simulink model "OPC_prueba_MPC_observador"  (R2018a)
settings: Solver=FixedStepAuto  StartTime=0.0  StopTime=inf  FixedStep=0.1  RelTol=1e-3
values from neighbouring files (symbols this model uses):
  Ad = sysd.A    [SimulinkInit.m]
  Bd = sysd.B    [SimulinkInit.m]
  Cd = sysd.C    [SimulinkInit.m]
libraries: opclib x7, mpclib x2
settings Model: Creator=cmparedes  LastModifiedBy=Diego
settings SolverCC: AutoInsertRateTranBlk=on

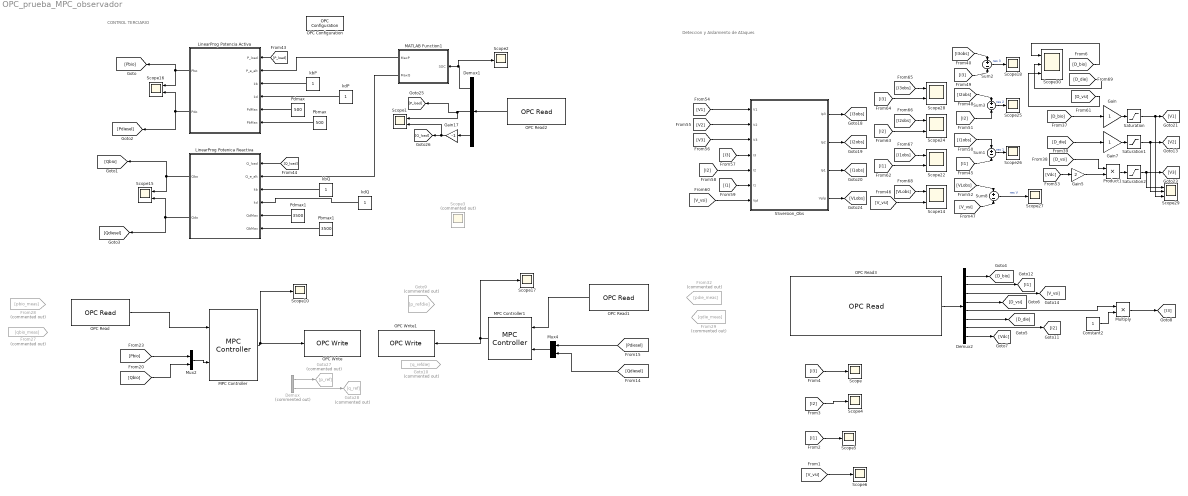
== system OPC_prueba_MPC_observador ==
  note: CONTROL TERCIARIO
  note: Deteccion y Aislamiento de Ataques
  Constant2 : Constant
  Demux : Demux  Commented=on  Outputs=2
  Demux1 : Demux  Outputs=3
  Demux2 : Demux  Outputs=8
  From27 : From  Commented=on  GotoTag=qbio_meas
  From28 : From  Commented=on  GotoTag=pbio_meas
  From29 : From  Commented=on  GotoTag=qdie_meas
  From32 : From  Commented=on  GotoTag=pdie_meas
  Gain : Gain
  Gain17 : Gain  Gain=-1
  Gain5 : Gain  Gain=2
  Gain7 : Gain
  Goto10 : Goto  Commented=on  GotoTag=q_refdie
  Goto27 : Goto  Commented=on  GotoTag=p_ref
  Goto28 : Goto  Commented=on  GotoTag=q_ref
  Goto9 : Goto  Commented=on  GotoTag=p_refdie
  LinearProg Potencia Activa : MATLAB Function  TreatAsAtomicUnit=on  SystemSampleTime=.1
  LinearProg Potenica Reactiva : MATLAB Function  TreatAsAtomicUnit=on  SystemSampleTime=.1
  MATLAB Function1 : MATLAB Function  TreatAsAtomicUnit=on
  MPC Controller : mpclib/MPC Controller  mpcobj=mpcobj  x0=[]  is_multiple=0  enable_value=0  return_u0=off  updateMPCinCallerWorkspace=on  ref_from_ws=off  ref_signal_name=[]  ref_preview=on  md_from_ws=off  md_signal_name=[]  md_preview=on  from_project=off  project_file=MPCtask.mat  md_inport=off  mv_inport=off  cost_outport=off  return_sequence=off  return_qpstatus=off  return_state=off  state_inport=off  lims_inport=off  cc_inport=off  ywt_inport=off  is_designfromscratch=0  uwt_inport=off  duwt_inport=off  rhoeps_inport=off  uref_inport=off  n_ts=0.1  n_p=100  n_mv=2  n_md=0  n_ud=0  n_mo=2  n_uo=0  BlockDataType=double  SampleTimeInherited=off  switch_inport=off
  MPC Controller1 : mpclib/MPC Controller  mpcobj=mpcobj  x0=[]  is_multiple=0  enable_value=0  return_u0=off  updateMPCinCallerWorkspace=on  ref_from_ws=off  ref_signal_name=[]  ref_preview=on  md_from_ws=off  md_signal_name=[]  md_preview=on  from_project=off  project_file=MPCtask.mat  md_inport=off  mv_inport=off  cost_outport=off  return_sequence=off  return_qpstatus=off  return_state=off  state_inport=off  lims_inport=off  cc_inport=off  ywt_inport=off  is_designfromscratch=0  uwt_inport=off  duwt_inport=off  rhoeps_inport=off  uref_inport=off  n_ts=0.1  n_p=100  n_mv=2  n_md=0  n_ud=0  n_mo=2  n_uo=0  BlockDataType=double  SampleTimeInherited=off  switch_inport=off
  Multiply : Product
  Mux2 : Mux  Inputs=2
  Mux4 : Mux  Inputs=2
  OPC Configuration : opclib/OPC Configuration  opcServers=localhost/Kepware.KEPServerEX.V6/10  errMissingItems=Error  errReadWrite=Warn  errShutdown=Error  errRTViolation=Warn  rtEnable=on  speedup=1  showLatency=off  beingUsed=on
      settings: SourceProductName=OPC Toolbox  SourceProductBaseCode=OT
  OPC Read : opclib/OPC Read  serverHost=localhost  serverID=Kepware.KEPServerEX.V6  itemIDs=BIO.Bio.Group1.Pm, BIO.Bio.Group1.Qm  readMode=Synchronous (device)  dataType=double  updateRate=0.1  showQual=off  showTS=off  tsMode=Seconds since start
      settings: SourceProductName=OPC Toolbox  SourceProductBaseCode=OT
  OPC Read1 : opclib/OPC Read  serverHost=localhost  serverID=Kepware.KEPServerEX.V6  itemIDs=EnergAlter.EnergAlter.Group1.Pm, EnergAlter.EnergAlter.Group1.Qm  readMode=Synchronous (device)  dataType=double  updateRate=0.1  showQual=off  showTS=off  tsMode=Seconds since start
      settings: SourceProductName=OPC Toolbox  SourceProductBaseCode=OT
  OPC Read2 : opclib/OPC Read  serverHost=localhost  serverID=Kepware.KEPServerEX.V6  itemIDs=EnergAlter.EnergAlter.Group1.SOC, Carga.Carga.Group1.Pm, Carga.Carga.Group1.Qm  readMode=Synchronous (device)  dataType=double  updateRate=0.1  showQual=off  showTS=off  tsMode=Seconds since start
      settings: SourceProductName=OPC Toolbox  SourceProductBaseCode=OT
  OPC Read3 : opclib/OPC Read  serverHost=localhost  serverID=Kepware.KEPServerEX.V6  itemIDs=BIO.Bio.Group1.duty_cycle1, BIO.Bio.Group1.Ibio, Carga.Carga.Group1.Vload, Diesel.Diesel.Group1.DieselDutyC, Diesel.Diesel.Group1.Idiesel, EnergAlter.EnergAlter.Group1.duty_cycle2, EnergAlter.EnergAlter.Group1.Ipv, Diesel.Diesel.Group1.DieselCaudal  readMode=Synchronous (device)  dataType=double  updateRate=0.1  showQual=off  showTS=off  tsMode=Seconds since start
      settings: SourceProductName=OPC Toolbox  SourceProductBaseCode=OT
  OPC Write : opclib/OPC Write  serverHost=localhost  serverID=Kepware.KEPServerEX.V6  itemIDs=BIO.Bio.Group1.Pref, BIO.Bio.Group1.Qref  writeMode=Synchronous  updateRate=0.1
      settings: SourceProductName=OPC Toolbox  SourceProductBaseCode=OT
  OPC Write1 : opclib/OPC Write  serverHost=localhost  serverID=Kepware.KEPServerEX.V6  itemIDs=EnergAlter.EnergAlter.Group1.Pref, EnergAlter.EnergAlter.Group1.Qref  writeMode=Synchronous  updateRate=0.1
      settings: SourceProductName=OPC Toolbox  SourceProductBaseCode=OT
  Pbmax : Constant  Value=500
  Pbmax1 : Constant  Value=3500
  Pdmax : Constant  Value=500
  Pdmax1 : Constant  Value=3500
  Product1 : Product
  SSversion_Obs : Subsystem
  Saturation : Saturate  UpperLimit=1000  LowerLimit=-1000
  Saturation1 : Saturate  UpperLimit=1000  LowerLimit=-1000
  Saturation2 : Saturate  UpperLimit=1000  LowerLimit=-1000
  Scope{,2,4..6,10,17..18,25..27} (11 alike) : Scope
  Scope{1,14..16,22,24,28} (7 alike) : Scope  NumInputPorts=2
  Scope29 : Scope  NumInputPorts=3
  Scope3 : Scope  Commented=on
  Scope30 : Scope  NumInputPorts=3
  Sum{1..3,8} (4 alike) : Sum  Inputs=+-
  kbP : Constant
  kbQ : Constant
  kdP : Constant
  kdQ : Constant
  wires:
  LinearProg Potencia Activa/1(Pbo) -> [Pbio], Scope16/1
  LinearProg Potencia Activa/2(Pdo) -> [Pdiesel], Scope16/2
  [Q_load] -> LinearProg Potenica Reactiva/1(Q_load)
  Pdmax1/1 -> LinearProg Potenica Reactiva/5(QdMax)
  kdP/1 -> LinearProg Potencia Activa/4(kd)
  [P_load] -> LinearProg Potencia Activa/1(P_load)
  LinearProg Potenica Reactiva/2(Qdo) -> Scope15/2, [Qdiesel]
  MATLAB Function1/2(MaxQ) -> LinearProg Potenica Reactiva/2(Q_e_alt)
  LinearProg Potenica Reactiva/1(Qbo) -> [Qbio], Scope15/1
  MATLAB Function1/1(MaxP) -> LinearProg Potencia Activa/2(P_e_alt)
  kdQ/1 -> LinearProg Potenica Reactiva/4(kd)
  kbP/1 -> LinearProg Potencia Activa/3(kb)
  kbQ/1 -> LinearProg Potenica Reactiva/3(kb)
  Pbmax/1 -> LinearProg Potencia Activa/6(PbMax)
  Pdmax/1 -> LinearProg Potencia Activa/5(PdMax)
  Gain17/1 -> Scope1/2, [Q_load]
  Pbmax1/1 -> LinearProg Potenica Reactiva/6(QbMax)
  OPC Read2/1 -> Demux1/1
  Demux1/1 -> Scope2/1, MATLAB Function1/1(SOC)
  Demux1/2 -> [P_load], Scope1/1
  MPC Controller1/1 -> OPC Write1/1, Scope17/1
  [Pbio] -> Mux2/1
  [Qbio] -> Mux2/2
  Demux/2 -> Goto28/1
  Demux/1 -> Goto27/1
  Mux2/1 -> MPC Controller/2
  MPC Controller/1 -> OPC Write/1, Scope10/1
  Mux4/1 -> MPC Controller1/2
  [Qdiesel] -> Mux4/2
  [Pdiesel] -> Mux4/1
  OPC Read1/1 -> MPC Controller1/1
  Demux1/3 -> Gain17/1
  OPC Read/1 -> MPC Controller/1
  [I2obs] -> Scope24/1
  [D_bio] -> Scope30/1
  Sum1/1 -> Scope26/1  "res 1"
  [D_die] -> Scope30/2
  [I2obs] -> Sum3/1
  [I1] -> Sum1/2
  [V_vsi] -> SSversion_Obs/7(Vpl)
  [I3] -> SSversion_Obs/4(I3)
  [Vdc] -> Gain5/1
  SSversion_Obs/1(Ip3) -> [I3obs]
  Saturation1/1 -> Scope29/2, [V2]
  [I3obs] -> Sum2/1
  [I2] -> SSversion_Obs/5(I2)
  [I2] -> Sum3/2
  SSversion_Obs/3(Ip1) -> [I1obs]
  [D_bio] -> Gain/1
  [I2] -> Scope24/2
  Product1/1 -> Saturation2/1
  [I1] -> Scope22/2
  [I3] -> Sum2/2
  [V1] -> SSversion_Obs/1(V1)
  [I3] -> Scope28/2
  [I3obs] -> Scope28/1
  [D_die] -> Gain7/1
  Saturation2/1 -> [V3], Scope29/1
  Saturation/1 -> [V1], Scope29/3
  [I1obs] -> Scope22/1
  Sum3/1 -> Scope25/1  "res 2"
  Gain7/1 -> Saturation1/1
  [VLobs] -> Sum8/1
  [I1obs] -> Sum1/1
  Sum8/1 -> Scope27/1  "res V"
  Gain5/1 -> Product1/2
  SSversion_Obs/2(Ip2) -> [I2obs]
  [I1] -> SSversion_Obs/6(I1)
  [D_vsi] -> Scope30/3
  Sum2/1 -> Scope18/1  "res 3"
  [V_vsi] -> Sum8/2
  [V2] -> SSversion_Obs/2(V2)
  [VLobs] -> Scope14/1
  [V3] -> SSversion_Obs/3(V3)
  SSversion_Obs/4(Vplp) -> [VLobs]
  [V_vsi] -> Scope14/2
  Gain/1 -> Saturation/1
  [D_vsi] -> Product1/1
  OPC Read3/1 -> Demux2/1
  Demux2/1 -> [D_bio]
  Demux2/6 -> [D_die]
  Demux2/4 -> [D_vsi]
  Demux2/2 -> [I1]
  Demux2/3 -> [V_vsi]
  Demux2/7 -> [I2]
  Demux2/8 -> [Vdc]
  Demux2/5 -> Multiply/1
  Constant2/1 -> Multiply/2
  Multiply/1 -> [I3]
  [I3] -> Scope/1
  [I2] -> Scope4/1
  [I1] -> Scope5/1
  [V_vsi] -> Scope6/1

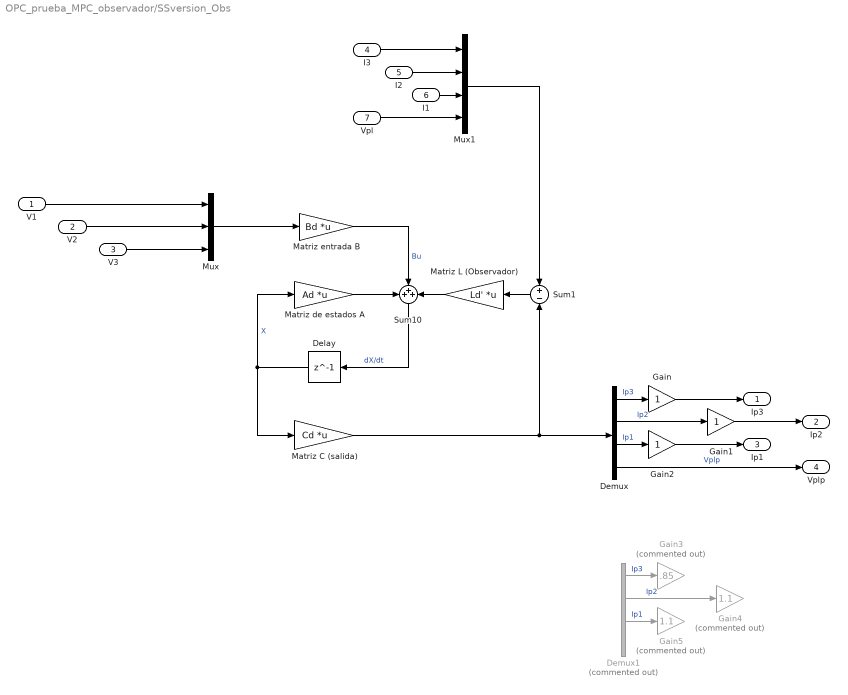
== system OPC_prueba_MPC_observador/SSversion_Obs ==
  V1 : Inport
  V2 : Inport  Port=2
  V3 : Inport  Port=3
  I3 : Inport  Port=4
  I2 : Inport  Port=5
  I1 : Inport  Port=6
  Vpl : Inport  Port=7
  Delay : Delay  DelayLength=1
  Demux : Demux
  Demux1 : Demux  Commented=on
  Gain : Gain
  Gain1 : Gain
  Gain2 : Gain
  Gain3 : Gain  Commented=on  Gain=.85
  Gain4 : Gain  Commented=on  Gain=1.1
  Gain5 : Gain  Commented=on  Gain=1.1
  Matriz C (salida) : Gain  Gain=Cd  Multiplication=Matrix(K*u)
  Matriz L (Observador) : Gain  Gain=Ld'  Multiplication=Matrix(K*u)
  Matriz de estados A : Gain  Gain=Ad  Multiplication=Matrix(K*u)
  Matriz entrada B : Gain  Gain=Bd  Multiplication=Matrix(K*u)
  Mux : Mux  Inputs=3
  Mux1 : Mux
  Sum1 : Sum  Inputs=+|-
  Sum10 : Sum  Inputs=+++
  Ip3 : Outport
  Ip2 : Outport  Port=2
  Ip1 : Outport  Port=3
  Vplp : Outport  Port=4
  wires:
  Matriz C (salida)/1 -> Demux/1, Sum1/2
  V1/1 -> Mux/1
  V2/1 -> Mux/2
  Demux/3 -> Gain2/1  "Ip1"
  V3/1 -> Mux/3
  Mux/1 -> Matriz entrada B/1
  Sum10/1 -> Delay/1  "dX/dt"
  Demux/2 -> Gain1/1  "Ip2"
  Demux/4 -> Vplp/1  "Vplp"
  Delay/1 -> Matriz de estados A/1, Matriz C (salida)/1  "X"
  Demux/1 -> Gain/1  "Ip3"
  Matriz de estados A/1 -> Sum10/1
  Matriz entrada B/1 -> Sum10/2  "Bu"
  I2/1 -> Mux1/2
  I3/1 -> Mux1/1
  I1/1 -> Mux1/3
  Vpl/1 -> Mux1/4
  Matriz L (Observador)/1 -> Sum10/3
  Sum1/1 -> Matriz L (Observador)/1
  Mux1/1 -> Sum1/1
  Gain/1 -> Ip3/1
  Gain1/1 -> Ip2/1
  Gain2/1 -> Ip1/1
  Demux1/1 -> Gain3/1  "Ip3"
  Demux1/2 -> Gain4/1  "Ip2"
  Demux1/3 -> Gain5/1  "Ip1"

== matlab function OPC_prueba_MPC_observador/LinearProg Potencia Activa ==
  data: P_load input; Pbo output; P_e_alt input; kb input; kd input; PdMax input; PbMax input; Pdo output
function [Pbo, Pdo] = fcn(P_load, P_e_alt, kb, kd, PdMax, PbMax)%, P_e_alt_min)

% P_load es la potencia que se requiere en la carga.

% P_e_alt es la potencia estimada de generacion de las energias
% alternativas

% kb y kd son los pesos de las funcion de costo.

% las salidas son las potencias optimas para bio y diesel

Pb=0;
Pd=0;

D_P_e_alt = P_e_alt %- P_e_alt_min % superaavit de energia alternativa.

flagDelt = 0;

if(D_P_e_alt >= P_load)
    flagDelt = 1;
end
   

if(flagDelt==0)
    P_trad = P_load - D_P_e_alt;
    % flag: variable que indica si tiene sentido evaluar los
    % if's que se encuentran mas adelante. es decir, si flag = 0 
    % despues del primer if entonces NO se le esta pidiendo al sistema
    % mas potencia de la que puede generar y portante el problema de 
    % optimizacion lineal tiene sentido.
    % entonces 
    flag=0;

    if(P_trad>PdMax+PbMax)
        Pd=PdMax;
        Pb=PbMax;
        flag=1;
    end

    % si ambas energias tienen el mismo factor de costo.
    if(kd==kb && flag==0)
        Pb=P_trad/2;
        Pd=P_trad/2;
    end

    % si la energia diesel es mas cara que la biomasa.
    if(kd>kb && flag==0)
        if(P_trad<=PbMax)
            Pb=P_trad;
            Pd=0;
        else
            Pb=PbMax;
            Pd=P_trad-PbMax;
        end
    end

    % si la biomasa es mas cara que la diesel.
    if(kd<kb && flag==0)
        if(P_trad<=PdMax)
            Pd=P_trad;
            Pb=0;
        else
            Pd=PdMax;
            Pb=P_trad-PdMax;
        end
    end
end

Pbo=Pb;
Pdo=Pd;

== matlab function OPC_prueba_MPC_observador/LinearProg Potenica Reactiva ==
  data: Q_load input; Qbo output; Q_e_alt input; kb input; kd input; QdMax input; QbMax input; Qdo output
function [Qbo, Qdo] = fcn(Q_load, Q_e_alt, kb, kd, QdMax, QbMax)

% Q_load es la potencia que se requiere en la carga.

% Q_e_alt es la potencia estimada de generacion de las energias
% alternativas

% kb y kd son los pesos de las funcion de costo.

% las salidas son las potencias optimas para bio y diesel

Qb=0;
Qd=0;

D_P_e_alt = Q_e_alt ;%- Q_e_alt_min % superaavit de energia alternativa.

flagDelt = 0;

if(D_P_e_alt >= Q_load)
    flagDelt = 1;
end
   

if(flagDelt==0)
    Q_trad = Q_load - D_P_e_alt;
    % flag: variable que indica si tiene sentido evaluar los
    % if's que se encuentran mas adelante. es decir, si flag = 0 
    % despues del primer if entonces NO se le esta pidiendo al sistema
    % mas potencia de la que puede generar y portante el problema de 
    % optimizacion lineal tiene sentido.
    % entonces 
    flag=0;

    if(Q_trad>QdMax+QbMax)
        Qd=QdMax;
        Qb=QbMax;
        flag=1;
    end

    % si ambas energias tienen el mismo factor de costo.
    if(kd==kb && flag==0)
        Qb=Q_trad/2;
        Qd=Q_trad/2;
    end

    % si la energia diesel es mas cara que la biomasa.
    if(kd>kb && flag==0)
        if(Q_trad<=QbMax)
            Qb=Q_trad;
            Qd=0;
        else
            Qb=QbMax;
            Qd=Q_trad-QbMax;
        end
    end

    % si la biomasa es mas cara que la diesel.
    if(kd<kb && flag==0)
        if(Q_trad<=QdMax)
            Qd=Q_trad;
            Qb=0;
        else
            Qd=QdMax;
            Qb=Q_trad-QdMax;
        end
    end
end

Qbo=Qb;
Qdo=Qd;

== matlab function OPC_prueba_MPC_observador/MATLAB Function1 ==
  data: SOC input; MaxP output; MaxQ output
function [MaxP, MaxQ] = fcn(SOC)


%  funcion que calcula la potencia maxima que puede suministrar las fuentes
%  renovables deacuerdo a la cantidad de carga que hay almancenada en la
%  bateria. esta va de 0 a 100%


% estoc valores que aparecen a continuacion se pusieron de manera
% arbitraria. corresponde a una persona con especialidad en la parte de
% potencia electrica determinar el verdadero algoritmo para hallar la
% potencia que deberia suministrar el nodo de energia renovable deacuerdo a
% la carga de la bateria.

MaxP = 0;
MaxQ = 0;

if( SOC >= 90 )
    MaxP = 500;
    MaxQ = 5000;
end

if( SOC <= 90 )
    MaxP = 200;
    MaxQ = 4000;
end

if( SOC <= 70 )
    MaxP = 100;
    MaxQ = 1000;
end

if( SOC <= 60 )
    MaxP = 50;
    MaxQ = 500;
end
